simulink model "TasksSimulink"  (R2017a)
settings: Solver=FixedStepAuto  StartTime=0.0  StopTime=time  FixedStep=0.01  RelTol=1e-3
values from neighbouring files (symbols this model uses):
  Cf = 81000    [Init_for_washout_filter.m]    (also in Task1c.m; UKF_start.m; workspace_updated.mat = 70000)
  Cr = 90000    [Init_for_washout_filter.m]    (also in Task1c.m; UKF_start.m; workspace_updated.mat = 80000)
  lf = 0.41*2.55    (= 1.0455)    [Init_for_washout_filter.m]    (also in UKF_start.m; workspace_updated.mat)
  lr = 2.55-lf    (= 1.5045)    [Init_for_washout_filter.m]    (also in UKF_start.m; workspace_updated.mat)
  mass = 1435-80    (= 1355)    [Init_for_washout_filter.m]    (also in UKF_start.m; workspace_updated.mat)
  Ratio = 17    [Init_for_washout_filter.m]    (also in UKF_start.m; workspace_updated.mat)
  rollGrad = 5*(pi/180)    (= 0.0872664625997)    [Init_for_washout_filter.m]    (also in UKF_start.m; workspace_updated.mat)
  rx = 0.4    [Init_for_washout_filter.m]    (also in UKF_start.m; workspace_updated.mat)
libraries: powerlib_meascontrol x2
settings Model: Creator=mitoa  LastModifiedBy=mitoa

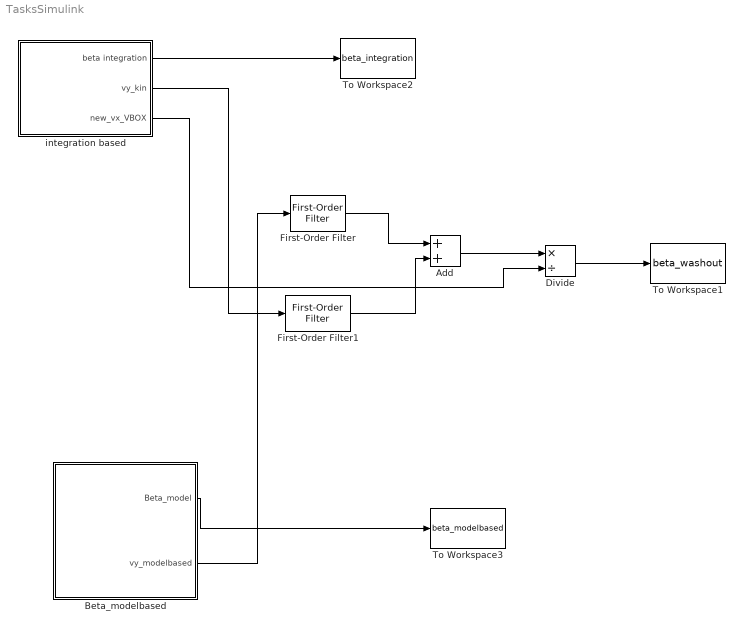
== system TasksSimulink ==
  Add : Sum
  Beta_modelbased : Subsystem
  Divide : Product  Inputs=*/
  First-Order Filter : powerlib_meascontrol/Filters/First-Order Filter  FilterType=Lowpass  Tc=T  Ts=0  Initialize=on  Vac_Init=[0, 0, 60]  Vdc_Init=0  PlotResponse=off  FreqRange="[0,  200,  1]"
      settings: SourceProductName=Simscape Power Systems
  First-Order Filter1 : powerlib_meascontrol/Filters/First-Order Filter  FilterType=Highpass  Tc=T  Ts=0  Initialize=on  Vac_Init=[0, 0, 60]  Vdc_Init=0  PlotResponse=off  FreqRange="[0,  200,  1]"
      settings: SourceProductName=Simscape Power Systems
  To Workspace1 : ToWorkspace  VariableName=beta_washout  SaveFormat=Timeseries  SampleTime=-1
  To Workspace2 : ToWorkspace  VariableName=beta_integration  SaveFormat=Timeseries  SampleTime=-1
  To Workspace3 : ToWorkspace  VariableName=beta_modelbased  SaveFormat=Timeseries  SampleTime=-1
  integration based : Subsystem
  wires:
  First-Order Filter/1 -> Add/1
  First-Order Filter1/1 -> Add/2
  Add/1 -> Divide/1
  integration based/3(new_vx_VBOX) -> Divide/2
  Divide/1 -> To Workspace1/1
  integration based/2(vy_kin) -> First-Order Filter1/1
  integration based/1(beta integration) -> To Workspace2/1
  Beta_modelbased/1(Beta_model) -> To Workspace3/1
  Beta_modelbased/2(vy_modelbased) -> First-Order Filter/1

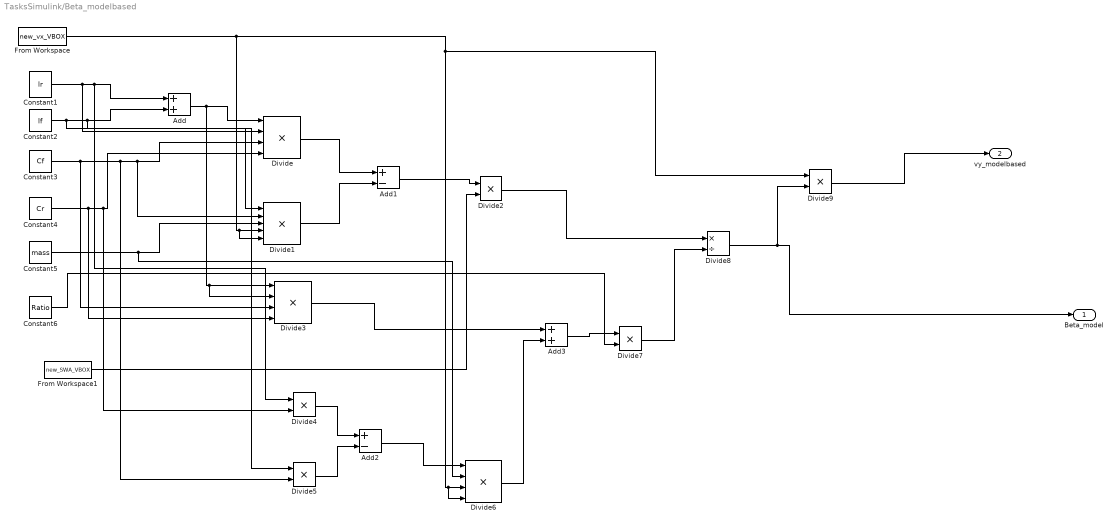
== system TasksSimulink/Beta_modelbased ==
  Add : Sum
  Add1 : Sum  Inputs=+-
  Add2 : Sum  Inputs=+-
  Add3 : Sum
  Constant1 : Constant  Value=lr
  Constant2 : Constant  Value=lf
  Constant3 : Constant  Value=Cf
  Constant4 : Constant  Value=Cr
  Constant5 : Constant  Value=mass
  Constant6 : Constant  Value=Ratio
  Divide : Product  Inputs=****
  Divide1 : Product  Inputs=*****
  Divide{2,4..5,7,9} (5 alike) : Product  Inputs=**
  Divide3 : Product  Inputs=****
  Divide6 : Product  Inputs=****
  Divide8 : Product  Inputs=*/
  From Workspace : FromWorkspace  VariableName=new_vx_VBOX  SampleTime=0
  From Workspace1 : FromWorkspace  VariableName=new_SWA_VBOX  SampleTime=0
  Beta_model : Outport
  vy_modelbased : Outport  Port=2
  wires:
  Constant2/1 -> Divide5/1, Divide1/1, Add/2
  Constant3/1 -> Divide3/3, Divide5/2, Divide1/2, Divide/3
  From Workspace/1 -> Divide9/1, Divide6/4, Divide6/3, Divide1/5, Divide1/4
  Constant1/1 -> Divide/2, Divide4/1, Add/1
  Constant4/1 -> Divide3/4, Divide4/2, Divide/4
  Add/1 -> Divide3/2, Divide3/1, Divide/1
  Divide/1 -> Add1/1
  Constant5/1 -> Divide6/2, Divide1/3
  Divide1/1 -> Add1/2
  Add1/1 -> Divide2/1
  Divide4/1 -> Add2/1
  Divide5/1 -> Add2/2
  Add2/1 -> Divide6/1
  Divide3/1 -> Add3/1
  Divide6/1 -> Add3/2
  Add3/1 -> Divide7/1
  Constant6/1 -> Divide7/2
  Divide2/1 -> Divide8/1
  Divide7/1 -> Divide8/2
  Divide8/1 -> Divide9/2, Beta_model/1
  From Workspace1/1 -> Divide2/2
  Divide9/1 -> vy_modelbased/1

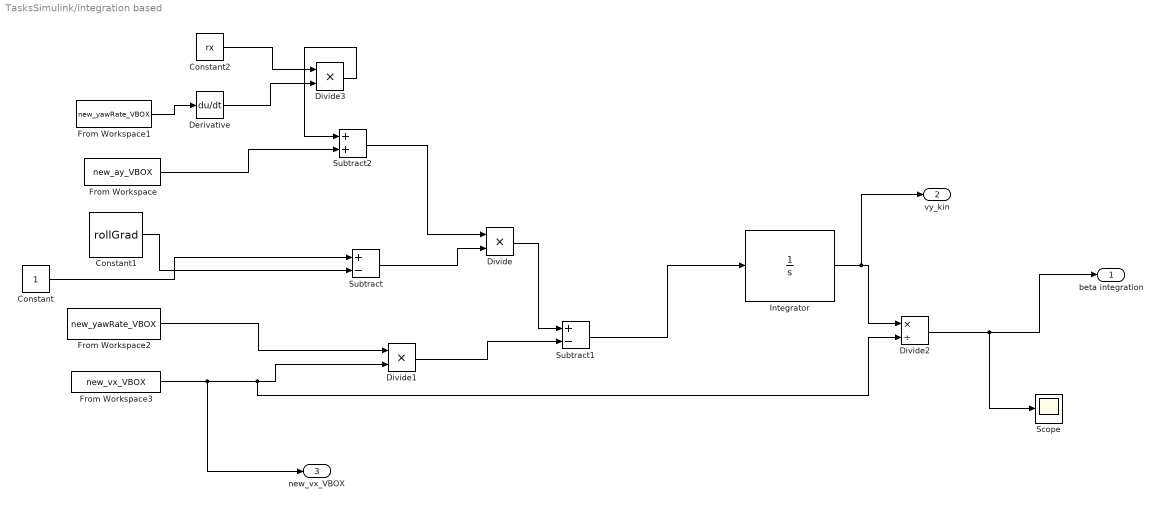
== system TasksSimulink/integration based ==
  Constant : Constant
  Constant1 : Constant  Value=rollGrad
  Constant2 : Constant  Value=rx
  Derivative : Derivative
  Divide : Product  Inputs=**
  Divide1 : Product  Inputs=**
  Divide2 : Product  Inputs=*/
  Divide3 : Product  Inputs=**
  From Workspace : FromWorkspace  VariableName=new_ay_VBOX  SampleTime=0
  From Workspace1 : FromWorkspace  VariableName=new_yawRate_VBOX  SampleTime=0
  From Workspace2 : FromWorkspace  VariableName=new_yawRate_VBOX  SampleTime=0
  From Workspace3 : FromWorkspace  VariableName=new_vx_VBOX  SampleTime=0
  Integrator : Integrator
  Scope : Scope
  Subtract : Sum  Inputs=+-
  Subtract1 : Sum  Inputs=+-
  Subtract2 : Sum
  beta integration : Outport
  vy_kin : Outport  Port=2
  new_vx_VBOX : Outport  Port=3
  wires:
  Constant/1 -> Subtract/1
  Divide2/1 -> beta integration/1, Scope/1
  Constant1/1 -> Subtract/2
  Subtract/1 -> Divide/2
  From Workspace3/1 -> new_vx_VBOX/1, Divide2/2, Divide1/2
  Subtract1/1 -> Integrator/1
  Divide/1 -> Subtract1/1
  Integrator/1 -> vy_kin/1, Divide2/1
  From Workspace2/1 -> Divide1/1
  Divide1/1 -> Subtract1/2
  From Workspace1/1 -> Derivative/1
  Constant2/1 -> Divide3/1
  Derivative/1 -> Divide3/2
  Divide3/1 -> Subtract2/1
  From Workspace/1 -> Subtract2/2
  Subtract2/1 -> Divide/1
